simulink model "TF_ex2"  (R2021b)
settings: Solver=VariableStepAuto  StartTime=0.0  StopTime=10.0  RelTol=1e-3
libraries: simulink x6
settings Model: Creator=Leonardo  LastModifiedBy=Leonardo

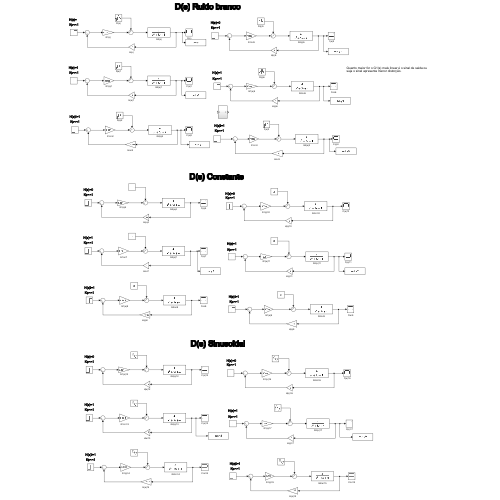
[thumbnail: Simulink's stored preview of the top-level diagram]
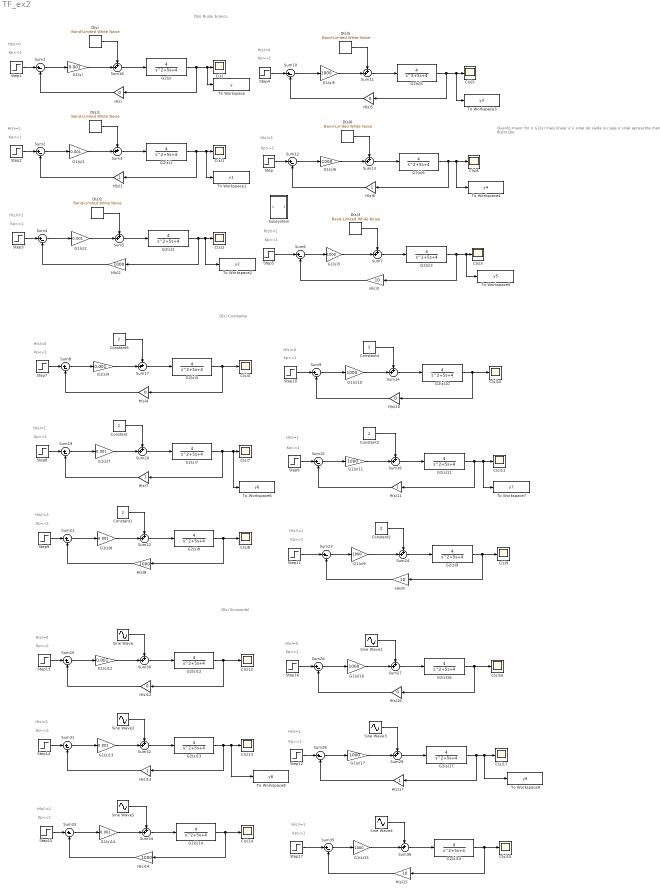
== system TF_ex2 ==
  note: H(s)!=1
  note: Kp>>1
  note: Kp>>1
  note: H(s)=0
  note: Kp<<1
  note: H(s)=0
  note: H(s)=0
  note: H(s)!=1
  note: Kp>>1
  note: H(s)=1
  note: H(s)!=1
  note: Kp>>1
  note: Kp<<1
  note: H(s)=1
  note: Kp>>1
  note: Kp<<1
  note: H(s)=1
  note: H(s)!=1
  note: Kp>>1
  note: H(s)=1
  note: H(s)=0
  note: Kp<<1
  note: D(s) Constante
  note: H(s)!=1
  note: H(s)=0
  note: D(s) Sinusoidal
  note: Kp<<1
  note: Kp>>1
  note: Kp<<1
  note: Kp<<1
  note: Kp<<1
  note: Quanto maior for o G1(s) mais linear é o sinal de saida ou seja o sinal apresenta menor distorção.
  note: Kp<<1
  note: H(s)!=1
  note: H(s)=0
  note: D(s) Ruido branco
  note: Kp>>1
  note: Kp>>1
  note: H(s)=1
  note: H(s)=1
  C(s){,1..17} (18 alike) : Scope
  Constant{,1..5} (6 alike) : Constant  Value=2
  D(s){,1..3,5..6} (6 alike) : simulink/Sources/Band-Limited White Noise  Cov=[0.01]  Ts=0.1  seed=[23341]
  G1(s){,1..2,4,7..8,12..14} (9 alike) : Gain  Gain=0.001
  G1(s){3,5..6,9..11,15..17} (9 alike) : Gain  Gain=1000
  G2(s){,1..17} (18 alike) : TransferFcn  Numerator=[4]  Denominator=[1 5 4]
  H(s){,4..5,10,12,16} (6 alike) : Gain  Gain=0
  H(s){1,6..7,11,13,17} (6 alike) : Gain
  H(s)14 : Gain  Gain=1000
  H(s)15 : Gain  Gain=10
  H(s)2 : Gain  Gain=1000
  H(s)3 : Gain  Gain=10
  H(s)8 : Gain  Gain=1000
  H(s)9 : Gain  Gain=10
  Sine Wave{,1..5} (6 alike) : Sin  SampleTime=0
  Step{,1..17} (18 alike) : Step  SampleTime=0
  Subsystem : Subsystem
  Sum{1..2,4,6,8..10,12,15,19,21,23,25..26,28,31,33,35} (18 alike) : Sum  Inputs=|+-
  Sum{3,5,7,11,13..14,16..18,20,22,24,27,29..30,32,34,36} (18 alike) : Sum  Inputs=++|
  To Workspace : ToWorkspace  VariableName=y  SaveFormat=Structure With Time  SampleTime=-1
  To Workspace1 : ToWorkspace  VariableName=y1  SaveFormat=Structure With Time  SampleTime=-1
  To Workspace2 : ToWorkspace  VariableName=y2  SaveFormat=Structure With Time  SampleTime=-1
  To Workspace3 : ToWorkspace  VariableName=y3  SaveFormat=Structure With Time  SampleTime=-1
  To Workspace4 : ToWorkspace  VariableName=y4  SaveFormat=Structure With Time  SampleTime=-1
  To Workspace5 : ToWorkspace  VariableName=y5  SaveFormat=Structure With Time  SampleTime=-1
  To Workspace6 : ToWorkspace  VariableName=y6  SaveFormat=Structure With Time  SampleTime=-1
  To Workspace7 : ToWorkspace  VariableName=y7  SaveFormat=Structure With Time  SampleTime=-1
  To Workspace8 : ToWorkspace  VariableName=y8  SaveFormat=Structure With Time  SampleTime=-1
  To Workspace9 : ToWorkspace  VariableName=y9  SaveFormat=Structure With Time  SampleTime=-1
  wires:
  G2(s)13/1 -> To Workspace8/1, C(s)13/1, H(s)13/1
  Sum9/1 -> G1(s)10/1
  G1(s)7/1 -> Sum20/2
  Sine Wave1/1 -> Sum27/1
  Constant/1 -> Sum20/1
  G1(s)14/1 -> Sum34/2
  Step11/1 -> Sum23/1
  H(s)14/1 -> Sum33/2
  G1(s)1/1 -> Sum3/2
  H(s)15/1 -> Sum35/2
  Step16/1 -> Sum26/1
  Sum19/1 -> G1(s)7/1
  H(s)13/1 -> Sum31/2
  G1(s)15/1 -> Sum36/2
  Sum16/1 -> G2(s)11/1
  Sum30/1 -> G2(s)12/1
  G2(s)3/1 -> To Workspace5/1, C(s)3/1, H(s)3/1
  Constant5/1 -> Sum17/1
  G2(s)9/1 -> C(s)9/1, H(s)9/1
  D(s)5/1 -> Sum11/1
  G2(s)6/1 -> H(s)6/1, To Workspace4/1, C(s)6/1
  Sum20/1 -> G2(s)7/1
  H(s)6/1 -> Sum12/2
  Step15/1 -> Sum33/1
  Step13/1 -> Sum25/1
  Sine Wave4/1 -> Sum36/1
  Sum22/1 -> G2(s)8/1
  Sum36/1 -> G2(s)15/1
  Sum33/1 -> G1(s)14/1
  Step4/1 -> Sum10/1
  H(s)4/1 -> Sum8/2
  D(s)6/1 -> Sum13/1
  Sum34/1 -> G2(s)14/1
  D(s)2/1 -> Sum5/1
  Sum35/1 -> G1(s)15/1
  Sum18/1 -> G2(s)/1
  H(s)8/1 -> Sum21/2
  Step14/1 -> Sum31/1
  G2(s)1/1 -> To Workspace1/1, C(s)1/1, H(s)1/1
  D(s)/1 -> Sum18/1
  D(s)1/1 -> Sum3/1
  G2(s)/1 -> To Workspace/1, C(s)/1, H(s)/1
  H(s)/1 -> Sum1/2
  G1(s)6/1 -> Sum13/2
  Step12/1 -> Sum28/1
  Step7/1 -> Sum8/1
  G2(s)5/1 -> To Workspace3/1, C(s)5/1, H(s)5/1
  Sum13/1 -> G2(s)6/1
  H(s)12/1 -> Sum25/2
  H(s)17/1 -> Sum28/2
  G2(s)17/1 -> H(s)17/1, To Workspace9/1, C(s)17/1
  H(s)16/1 -> Sum26/2
  G2(s)12/1 -> C(s)12/1, H(s)12/1
  G1(s)17/1 -> Sum29/2
  D(s)3/1 -> Sum7/1
  G2(s)15/1 -> C(s)15/1, H(s)15/1
  Sum5/1 -> G2(s)2/1
  Sum27/1 -> G2(s)16/1
  G2(s)2/1 -> To Workspace2/1, C(s)2/1, H(s)2/1
  H(s)7/1 -> Sum19/2
  G1(s)8/1 -> Sum22/2
  G1(s)4/1 -> Sum17/2
  Step6/1 -> Sum15/1
  Constant3/1 -> Sum16/1
  Sum3/1 -> G2(s)1/1
  Constant4/1 -> Sum14/1
  Step10/1 -> Sum9/1
  G1(s)3/1 -> Sum7/2
  Sum7/1 -> G2(s)3/1
  Sum6/1 -> G1(s)3/1
  Step5/1 -> Sum6/1
  Step1/1 -> Sum1/1
  Sum24/1 -> G2(s)9/1
  Sum28/1 -> G1(s)17/1
  H(s)1/1 -> Sum2/2
  Constant2/1 -> Sum24/1
  G1(s)2/1 -> Sum5/2
  Sum1/1 -> G1(s)/1
  G1(s)/1 -> Sum18/2
  Sum10/1 -> G1(s)5/1
  Constant1/1 -> Sum22/1
  G2(s)10/1 -> C(s)10/1, H(s)10/1
  Step2/1 -> Sum2/1
  G2(s)4/1 -> C(s)4/1, H(s)4/1
  Sum32/1 -> G2(s)13/1
  G1(s)9/1 -> Sum24/2
  H(s)10/1 -> Sum9/2
  H(s)5/1 -> Sum10/2
  G1(s)5/1 -> Sum11/2
  Step9/1 -> Sum21/1
  Step3/1 -> Sum4/1
  G2(s)7/1 -> To Workspace6/1, C(s)7/1, H(s)7/1
  G2(s)8/1 -> C(s)8/1, H(s)8/1
  G2(s)16/1 -> C(s)16/1, H(s)16/1
  Sum11/1 -> G2(s)5/1
  Step17/1 -> Sum35/1
  Step/1 -> Sum12/1
  H(s)11/1 -> Sum15/2
  G1(s)11/1 -> Sum16/2
  H(s)3/1 -> Sum6/2
  G2(s)11/1 -> H(s)11/1, To Workspace7/1, C(s)11/1
  H(s)9/1 -> Sum23/2
  Sum29/1 -> G2(s)17/1
  G1(s)12/1 -> Sum30/2
  G2(s)14/1 -> C(s)14/1, H(s)14/1
  Sum2/1 -> G1(s)1/1
  Sum12/1 -> G1(s)6/1
  Sum4/1 -> G1(s)2/1
  Sum25/1 -> G1(s)12/1
  Sum31/1 -> G1(s)13/1
  Sum23/1 -> G1(s)9/1
  H(s)2/1 -> Sum4/2
  Sum14/1 -> G2(s)10/1
  G1(s)13/1 -> Sum32/2
  Sum17/1 -> G2(s)4/1
  Sum15/1 -> G1(s)11/1
  Sine Wave2/1 -> Sum32/1
  Sum26/1 -> G1(s)16/1
  Sine Wave3/1 -> Sum29/1
  G1(s)16/1 -> Sum27/2
  Step8/1 -> Sum19/1
  G1(s)10/1 -> Sum14/2
  Sine Wave5/1 -> Sum34/1
  Sine Wave/1 -> Sum30/1
  Sum21/1 -> G1(s)8/1
  Sum8/1 -> G1(s)4/1

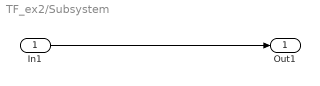
== system TF_ex2/Subsystem ==
  In1 : Inport
  Out1 : Outport
  wires:
  In1/1 -> Out1/1
